simulink model "sysgenConcatenatedFEC"  (Simulink 7.4)
settings: Solver=ode45  SolverMode=SingleTasking  StartTime=0.0  StopTime=5000  RelTol=1e-3
undefined symbols (not defined in the file or in its folder): De, Interleaver, interleaver
libraries: xbsIndex_r4 x119, commchan3 x2, commdigbbndpm3 x2, xbsCopyrightNotice_r4 x1
(part 2 of 2)

== system sysgenConcatenatedFEC/Encoder1/rsenc ==
  note: The Outer Encoder is implemented by selecting  the RS Encoder block in the Xilinx Communication library. The
      | RS Encoder block has a pull down option to implement the DVB specifications specified in the standard. The
      | Reinterpret1 block at the input of the RS encoder converts the input FIX8_6 to UFIX8_0. The rfd output from the RS
      | Encoder block is used for handshaking to avoid any input data being dropped when the RS Encoder is generating
      | parity symbols.The RS Encoder block synchronizes its output to the first valid data received at the input.
  din : Inport  OutDataType=sfix(16)  OutScaling=2^0
  Constant : xbsIndex_r4/Constant  arith_type=Boolean  const=1  n_bits=1  bin_pt=0  explicit_period=on  period=1  equ=P=C  opselect=C  inp2=PCIN>>17  opr=+  inp1=P  carry=CIN  dbl_ovrd=off  block_type=constant
      settings: block_version=VER_STRING_GOES_HERE
  Delay : xbsIndex_r4/Delay  en=off  latency=2  dbl_ovrd=off  reg_retiming=off  block_type=delay
      settings: infoedit="Delay line having  configurable length.<P><P>Hardware notes: A delay line is a chain, each link of which is an SRL16 followed by a flip-flop. If register retiming is enabled, the delay line is a chain of flip-flops."  xl_area=[0, 0, 0, 0, 0, 0, 0]  block_version=VER_STRING_GOES_HERE
  RS Encoder : Subsystem
      settings: CopyFcn=set_param(gcb, 'LinkStatus', 'none');
  Reinterpret : xbsIndex_r4/Reinterpret  force_arith_type=on  arith_type=Unsigned  force_bin_pt=on  bin_pt=0  block_type=cast
      settings: infoedit="Changes type of samples without altering their binary representation.<P><P>Hardware notes: In hardware this block costs nothing.<P><P>Example:  Suppose the input is 6 bits wide, signed, with 2 fractional bits, and the output is forced to unsigned with 0 fractional bits.  Then an input of -2.0 (1110.00 in binary 2's complement) becomes an output of 56 (111000 in binary)."  block_version=VER_STRING_GOES_HERE
  tmt : Terminator
  dout : Outport  OutDataType=sfix(16)  OutScaling=2^0
  vout : Outport  Port=2  OutDataType=sfix(16)  OutScaling=2^0
  rfd : Outport  Port=3  OutDataType=sfix(16)  OutScaling=2^0
  wires:
  Constant/1 -> Delay/1
  Delay/1 -> RS Encoder/2(vin)
  RS Encoder/2(vout) -> vout/1
  RS Encoder/3(info) -> tmt/1
  RS Encoder/4(rfd) -> rfd/1
  Reinterpret/1 -> RS Encoder/1(din)
  din/1 -> Reinterpret/1
  RS Encoder/1(dout) -> dout/1

== system sysgenConcatenatedFEC/Decoder1/cvdeint/Rising Edge Detector1 ==
  Din : Inport  OutDataType=sfix(16)  OutScaling=2^0
  Delay : xbsIndex_r4/Delay  en=off  latency=1  dbl_ovrd=off  reg_retiming=off  block_type=delay
      settings: block_version=12.1
  Inverter2 : xbsIndex_r4/Inverter  en=off  latency=0  dbl_ovrd=off  block_type=inv
      settings: block_version=9.1
  Logical : xbsIndex_r4/Logical  logical_function=AND  inputs=2  en=off  latency=0  precision=Full  arith_type=Unsigned  n_bits=16  bin_pt=0  align_bp=on  dbl_ovrd=off  block_type=logical
      settings: block_version=9.1
  Register1 : xbsIndex_r4/Register  init=0  rst=off  en=off  dbl_ovrd=off  block_type=register
      settings: block_version=9.1
  Dout : Outport  OutDataType=sfix(16)  OutScaling=2^0
  wires:
  Delay/1 -> Dout/1
  Inverter2/1 -> Logical/2
  Register1/1 -> Inverter2/1
  Din/1 -> Logical/1, Register1/1
  Logical/1 -> Delay/1

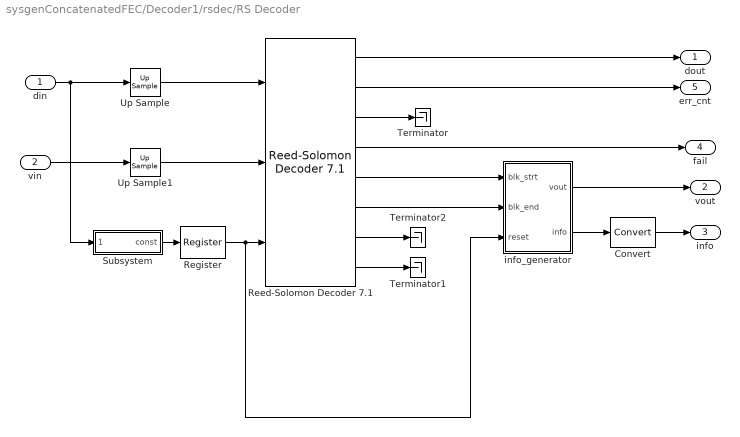
== system sysgenConcatenatedFEC/Decoder1/rsdec/RS Decoder ==
  din : Inport  OutDataType=sfix(16)  OutScaling=2^0
  vin : Inport  Port=2  OutDataType=sfix(16)  OutScaling=2^0
  Convert : xbsIndex_r4/Convert  arith_type=Boolean  n_bits=8  bin_pt=6  quantization=Truncate  overflow=Wrap  en=off  latency=0  dbl_ovrd=off  pipeline=off  block_type=convert
      settings: infoedit=The input is presented at the output after quantization and overflow effects.<P><P>Hardware notes: Additional hardware is used when rounding or saturation is selected and output width is less than the input width.  block_version=VER_STRING_GOES_HERE
  "Reed-Solomon Decoder 7.1 " : xbsIndex_r4/Reed-Solomon Decoder 7.1   code_specification=DVB  symbol_width=8  field_polynomial=285  scaling_factor=1  generator_start=0  variable_block_length=off  symbols_per_block=204  data_symbols=188  variable_number_of_check_symbols=off  define_supported_r_in_values=off  number_of_supported_r_in_values=2  supported_r_in_definition_file='no_coe_file_loaded'  optimization=Speed  self_recovering=off  memory_style=Automatic  clocks_per_symbol=8  number_of_channels=1  number_of_puncture_patterns=0  puncture_definition_file='no_coe_file_loaded'  clock_enable=off  info_end=off  synchronous_reset=on  original_delayed_data=off  erase=off  error_statistics=off  marker_bits=off  number_of_marker_bits=1  ip_name=Reed-Solomon Decoder  ip_version=7.1  dsptool_ready=false  ipcore_usecache=true  ipcore_useipmodelcache=true  wrapper_available=true  port_translation_map={ 'ce' => 'en', 'sr' => 'rst'}  structural_sim=true  ipcore_do_not_force_period=true  block_type=rs_decoder_v7_1
      settings: block_version=12.2
  Register : xbsIndex_r4/Register  init=0  rst=off  en=off  dbl_ovrd=off  block_type=register
      settings: block_version=12.1
  Subsystem : Subsystem
  Terminator : Terminator
  Terminator1 : Terminator
  Terminator2 : Terminator
  Up Sample : xbsIndex_r4/Up Sample  sample_ratio=8  copy_samples=on  en=off  latency=0  dbl_ovrd=off  block_type=usamp
      settings: block_version=12.1
  Up Sample1 : xbsIndex_r4/Up Sample  sample_ratio=8  copy_samples=on  en=off  latency=0  dbl_ovrd=off  block_type=usamp
      settings: block_version=12.1
  info_generator : Subsystem  mask{sym_width=8, kk=188}
      mask prompts: sym_width "Symbol Width"; kk "Number of information symbols per code block"
  dout : Outport  OutDataType=sfix(16)  OutScaling=2^0
  vout : Outport  Port=2  OutDataType=sfix(16)  OutScaling=2^0
  info : Outport  Port=3  OutDataType=sfix(16)  OutScaling=2^0
  fail : Outport  Port=4  OutDataType=sfix(16)  OutScaling=2^0
  err_cnt : Outport  Port=5  OutDataType=sfix(16)  OutScaling=2^0
  wires:
  "Reed-Solomon Decoder 7.1 "/7 -> Terminator2/1
  "Reed-Solomon Decoder 7.1 "/8 -> Terminator1/1
  "Reed-Solomon Decoder 7.1 "/3 -> Terminator/1
  "Reed-Solomon Decoder 7.1 "/4 -> fail/1
  "Reed-Solomon Decoder 7.1 "/2 -> err_cnt/1
  Convert/1 -> info/1
  Subsystem/1(const) -> Register/1
  din/1 -> Subsystem/1(sample), Up Sample/1
  vin/1 -> Up Sample1/1
  "Reed-Solomon Decoder 7.1 "/1 -> dout/1
  "Reed-Solomon Decoder 7.1 "/6 -> info_generator/2(blk_end)
  "Reed-Solomon Decoder 7.1 "/5 -> info_generator/1(blk_strt)
  info_generator/1(vout) -> vout/1
  info_generator/2(info) -> Convert/1
  Up Sample/1 -> "Reed-Solomon Decoder 7.1 "/1
  Up Sample1/1 -> "Reed-Solomon Decoder 7.1 "/2
  Register/1 -> info_generator/3(reset), "Reed-Solomon Decoder 7.1 "/3

== system sysgenConcatenatedFEC/Encoder1/int/Rising Edge Detector1 ==
  Din : Inport  OutDataType=sfix(16)  OutScaling=2^0
  Delay : xbsIndex_r4/Delay  en=off  latency=1  dbl_ovrd=off  reg_retiming=off  block_type=delay
      settings: block_version=12.1
  Inverter2 : xbsIndex_r4/Inverter  en=off  latency=0  dbl_ovrd=off  block_type=inv
      settings: block_version=9.1
  Logical : xbsIndex_r4/Logical  logical_function=AND  inputs=2  en=off  latency=0  precision=Full  arith_type=Unsigned  n_bits=16  bin_pt=0  align_bp=on  dbl_ovrd=off  block_type=logical
      settings: block_version=9.1
  Register1 : xbsIndex_r4/Register  init=0  rst=off  en=off  dbl_ovrd=off  block_type=register
      settings: block_version=9.1
  Dout : Outport  OutDataType=sfix(16)  OutScaling=2^0
  wires:
  Delay/1 -> Dout/1
  Inverter2/1 -> Logical/2
  Register1/1 -> Inverter2/1
  Din/1 -> Logical/1, Register1/1
  Logical/1 -> Delay/1

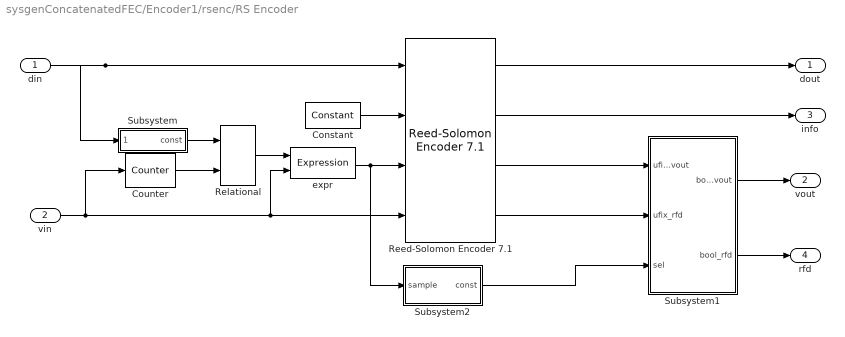
== system sysgenConcatenatedFEC/Encoder1/rsenc/RS Encoder ==
  din : Inport  OutDataType=sfix(16)  OutScaling=2^0
  vin : Inport  Port=2  OutDataType=sfix(16)  OutScaling=2^0
  Constant : xbsIndex_r4/Constant  arith_type=Boolean  const=0  n_bits=1  bin_pt=0  explicit_period=off  period=1  equ=P=C  opselect=C  inp2=PCIN>>17  opr=+  inp1=P  carry=CIN  dbl_ovrd=off  block_type=constant
      settings: block_version=VER_STRING_GOES_HERE
  Counter : xbsIndex_r4/Counter  cnt_type=Count Limited  cnt_to=204-1  operation=Up  start_count=0  cnt_by_val=1  arith_type=Unsigned  n_bits=8  bin_pt=0  load_pin=off  rst=off  en=on  explicit_period=off  period=1  dbl_ovrd=off  use_behavioral_HDL=off  implementation=Fabric  use_rpm=off  block_type=counter
      settings: infoedit="Configurable up, down and up/down counter.<P><P>Hardware notes: Free running counters are the least expensive in hardware.  A count limited counter is implemented by combining a counter with a comparator."  block_version=VER_STRING_GOES_HERE
  "Reed-Solomon Encoder 7.1 " : xbsIndex_r4/Reed-Solomon Encoder 7.1   code_specification=DVB  variable_number_of_check_symbols=off  variable_block_length=off  symbol_width=8  field_polynomial=285  scaling_factor=1  generator_start=0  symbol_per_block=204  data_symbols=188  check_symbol_generator=Fixed_Architecture  memory_style=Automatic  number_of_channels=1  ce=off  rdy=on  nd=on  rfd=on  sclr=off  rffd=off  ip_name=Reed-Solomon Encoder  ip_version=7.1  dsptool_ready=false  ipcore_usecache=true  ipcore_useipmodelcache=true  wrapper_available=true  port_translation_map={ 'ce' => 'en', 'sclr' => 'rst'}  structural_sim=false  ipcore_do_not_force_period=true  block_type=rs_encoder_v7_1
      settings: block_version=12.2
  Relational : xbsIndex_r4/Relational  mode=a=b  en=off  latency=0  dbl_ovrd=off  block_type=relational
      settings: block_version=VER_STRING_GOES_HERE
  Subsystem : Subsystem
  Subsystem1 : Subsystem
  Subsystem2 : Subsystem
  expr : xbsIndex_r4/Expression  expression=a & b  align_bp=on  en=off  latency=0  precision=Full  arith_type=Unsigned  n_bits=8  bin_pt=2  dbl_ovrd=off  block_type=expr
      settings: block_version=VER_STRING_GOES_HERE
  dout : Outport  OutDataType=sfix(16)  OutScaling=2^0
  vout : Outport  Port=2  OutDataType=sfix(16)  OutScaling=2^0
  info : Outport  Port=3  OutDataType=sfix(16)  OutScaling=2^0
  rfd : Outport  Port=4  OutDataType=sfix(16)  OutScaling=2^0
  wires:
  Subsystem2/1(const) -> Subsystem1/3(sel)
  din/1 -> Subsystem/1(sample), "Reed-Solomon Encoder 7.1 "/1
  "Reed-Solomon Encoder 7.1 "/1 -> dout/1
  "Reed-Solomon Encoder 7.1 "/2 -> info/1
  Constant/1 -> "Reed-Solomon Encoder 7.1 "/2
  vin/1 -> Counter/1, expr/2, "Reed-Solomon Encoder 7.1 "/4
  expr/1 -> Subsystem2/1(sample), "Reed-Solomon Encoder 7.1 "/3
  Relational/1 -> expr/1
  Counter/1 -> Relational/2
  "Reed-Solomon Encoder 7.1 "/3 -> Subsystem1/1(ufix_vout)
  "Reed-Solomon Encoder 7.1 "/4 -> Subsystem1/2(ufix_rfd)
  Subsystem1/2(bool_rfd) -> rfd/1
  Subsystem/1(const) -> Relational/1
  Subsystem1/1(bool_vout) -> vout/1

== system sysgenConcatenatedFEC/Decoder1/rsdec/RS Decoder/Subsystem ==
  sample : Inport  OutDataType=sfix(16)  OutScaling=2^0
  Constant4 : xbsIndex_r4/Constant  arith_type=Boolean  const=0  n_bits=1  bin_pt=0  explicit_period=off  period=1  equ=P=C  opselect=C  inp2=PCIN>>17  opr=+  inp1=P  carry=CIN  dbl_ovrd=off  block_type=constant
      settings: block_version=VER_STRING_GOES_HERE
  Slice : xbsIndex_r4/Slice  nbits=1  boolean_output=on  mode=Upper Bit Location + Width  bit1=0  base1=MSB of Input  bit0=0  base0=LSB of Input  dbl_ovrd=off  block_type=slice
      settings: infoedit="Extracts a given range of bits from each input sample and presents it at the output.  The output type is ordinarily unsigned with binary point at zero, but can be Boolean when the slice is one bit wide.<P><P>Hardware notes: In hardware this block costs nothing."  block_version=VER_STRING_GOES_HERE
  expr2 : xbsIndex_r4/Expression  expression=a & b  align_bp=on  en=off  latency=0  precision=Full  arith_type=Unsigned  n_bits=8  bin_pt=2  dbl_ovrd=off  block_type=expr
      settings: block_version=VER_STRING_GOES_HERE
  const : Outport  OutDataType=sfix(16)  OutScaling=2^0
  wires:
  expr2/1 -> const/1
  sample/1 -> Slice/1
  Slice/1 -> expr2/1
  Constant4/1 -> expr2/2

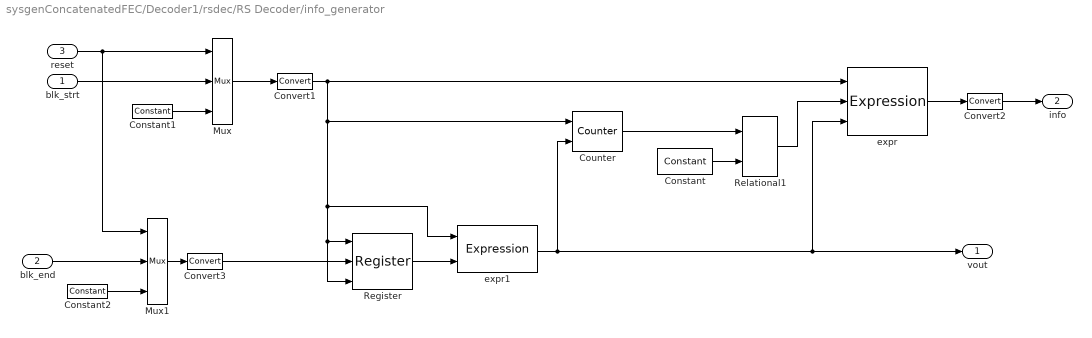
== system sysgenConcatenatedFEC/Decoder1/rsdec/RS Decoder/info_generator ==
  blk_strt : Inport  OutDataType=sfix(16)  OutScaling=2^0
  blk_end : Inport  Port=2  OutDataType=sfix(16)  OutScaling=2^0
  reset : Inport  Port=3  OutDataType=sfix(16)  OutScaling=2^0
  Constant : xbsIndex_r4/Constant  arith_type=Unsigned  const=kk-1  n_bits=8  bin_pt=0  explicit_period=off  period=1  equ=P=C  opselect=C  inp2=PCIN>>17  opr=+  inp1=P  carry=CIN  dbl_ovrd=off  block_type=constant
      settings: block_version=VER_STRING_GOES_HERE
  Constant1 : xbsIndex_r4/Constant  arith_type=Boolean  const=0  n_bits=1  bin_pt=0  explicit_period=off  period=1  equ=P=C  opselect=C  inp2=PCIN>>17  opr=+  inp1=P  carry=CIN  dbl_ovrd=off  block_type=constant
      settings: block_version=VER_STRING_GOES_HERE
  Constant2 : xbsIndex_r4/Constant  arith_type=Boolean  const=0  n_bits=1  bin_pt=0  explicit_period=off  period=1  equ=P=C  opselect=C  inp2=PCIN>>17  opr=+  inp1=P  carry=CIN  dbl_ovrd=off  block_type=constant
      settings: block_version=VER_STRING_GOES_HERE
  Convert1 : xbsIndex_r4/Convert  arith_type=Boolean  n_bits=1  bin_pt=0  quantization=Truncate  overflow=Wrap  en=off  latency=0  dbl_ovrd=off  pipeline=off  block_type=convert
      settings: infoedit=The input is presented at the output after quantization and overflow effects.<P><P>Hardware notes: Additional hardware is used when rounding or saturation is selected and output width is less than the input width.  block_version=VER_STRING_GOES_HERE
  Convert2 : xbsIndex_r4/Convert  arith_type=Unsigned  n_bits=1  bin_pt=0  quantization=Truncate  overflow=Wrap  en=off  latency=0  dbl_ovrd=off  pipeline=off  block_type=convert
      settings: infoedit=The input is presented at the output after quantization and overflow effects.<P><P>Hardware notes: Additional hardware is used when rounding or saturation is selected and output width is less than the input width.  block_version=VER_STRING_GOES_HERE
  Convert3 : xbsIndex_r4/Convert  arith_type=Boolean  n_bits=1  bin_pt=0  quantization=Truncate  overflow=Wrap  en=off  latency=0  dbl_ovrd=off  pipeline=off  block_type=convert
      settings: infoedit=The input is presented at the output after quantization and overflow effects.<P><P>Hardware notes: Additional hardware is used when rounding or saturation is selected and output width is less than the input width.  block_version=VER_STRING_GOES_HERE
  Counter : xbsIndex_r4/Counter  cnt_type=Free Running  cnt_to=inf  operation=Up  start_count=0  cnt_by_val=1  arith_type=Unsigned  n_bits=sym_width  bin_pt=0  load_pin=off  rst=on  en=on  explicit_period=off  period=1  dbl_ovrd=off  use_behavioral_HDL=off  implementation=Fabric  use_rpm=off  block_type=counter
      settings: infoedit="Configurable up, down and up/down counter.<P><P>Hardware notes: Free running counters are the least expensive in hardware.  A count limited counter is implemented by combining a counter with a comparator."  block_version=VER_STRING_GOES_HERE
  Mux : xbsIndex_r4/Mux  inputs=2  en=off  latency=0  precision=Full  arith_type=Unsigned  n_bits=8  bin_pt=2  quantization=Truncate  overflow=Wrap  dbl_ovrd=off  block_type=mux
      settings: block_version=VER_STRING_GOES_HERE
  Mux1 : xbsIndex_r4/Mux  inputs=2  en=off  latency=0  precision=Full  arith_type=Unsigned  n_bits=8  bin_pt=2  quantization=Truncate  overflow=Wrap  dbl_ovrd=off  block_type=mux
      settings: block_version=VER_STRING_GOES_HERE
  Register : xbsIndex_r4/Register  init=0  rst=on  en=on  dbl_ovrd=off  block_type=register
      settings: block_version=VER_STRING_GOES_HERE
  Relational1 : xbsIndex_r4/Relational  mode=a<b  en=off  latency=0  dbl_ovrd=off  block_type=relational
      settings: block_version=VER_STRING_GOES_HERE
  expr : xbsIndex_r4/Expression  expression=(a | b) & c  align_bp=on  en=off  latency=0  precision=Full  arith_type=Unsigned  n_bits=8  bin_pt=2  dbl_ovrd=off  block_type=expr
      settings: block_version=VER_STRING_GOES_HERE
  expr1 : xbsIndex_r4/Expression  expression=a | b  align_bp=on  en=off  latency=0  precision=Full  arith_type=Unsigned  n_bits=8  bin_pt=2  dbl_ovrd=off  block_type=expr
      settings: block_version=VER_STRING_GOES_HERE
  vout : Outport  OutDataType=sfix(16)  OutScaling=2^0
  info : Outport  Port=2  OutDataType=sfix(16)  OutScaling=2^0
  wires:
  Convert3/1 -> Register/2
  Constant/1 -> Relational1/2
  Relational1/1 -> expr/2
  Counter/1 -> Relational1/1
  Convert1/1 -> expr/1, Counter/1, Register/1, Register/3, expr1/1
  expr/1 -> Convert2/1
  Convert2/1 -> info/1
  Mux/1 -> Convert1/1
  Constant1/1 -> Mux/3
  blk_strt/1 -> Mux/2
  reset/1 -> Mux/1, Mux1/1
  Mux1/1 -> Convert3/1
  Constant2/1 -> Mux1/3
  blk_end/1 -> Mux1/2
  Register/1 -> expr1/2
  expr1/1 -> expr/3, vout/1, Counter/2

== system sysgenConcatenatedFEC/Encoder1/rsenc/RS Encoder/Subsystem ==
  sample : Inport  OutDataType=sfix(16)  OutScaling=2^0
  Constant4 : xbsIndex_r4/Constant  arith_type=Unsigned  const=0  n_bits=1  bin_pt=0  explicit_period=off  period=1  equ=P=C  opselect=C  inp2=PCIN>>17  opr=+  inp1=P  carry=CIN  dbl_ovrd=off  block_type=constant
      settings: block_version=VER_STRING_GOES_HERE
  Slice : xbsIndex_r4/Slice  nbits=1  boolean_output=off  mode=Upper Bit Location + Width  bit1=0  base1=MSB of Input  bit0=0  base0=LSB of Input  dbl_ovrd=off  block_type=slice
      settings: infoedit="Extracts a given range of bits from each input sample and presents it at the output.  The output type is ordinarily unsigned with binary point at zero, but can be Boolean when the slice is one bit wide.<P><P>Hardware notes: In hardware this block costs nothing."  block_version=VER_STRING_GOES_HERE
  expr2 : xbsIndex_r4/Expression  expression=a & b  align_bp=on  en=off  latency=0  precision=Full  arith_type=Unsigned  n_bits=8  bin_pt=2  dbl_ovrd=off  block_type=expr
      settings: block_version=VER_STRING_GOES_HERE
  const : Outport  OutDataType=sfix(16)  OutScaling=2^0
  wires:
  Constant4/1 -> expr2/2
  Slice/1 -> expr2/1
  sample/1 -> Slice/1
  expr2/1 -> const/1

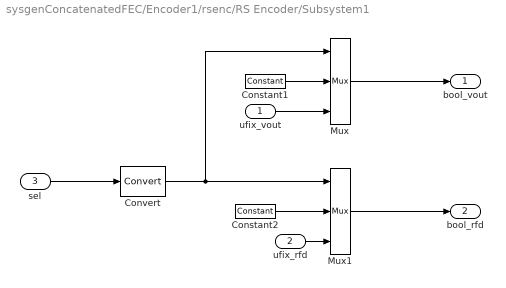
== system sysgenConcatenatedFEC/Encoder1/rsenc/RS Encoder/Subsystem1 ==
  ufix_vout : Inport  OutDataType=sfix(16)  OutScaling=2^0
  ufix_rfd : Inport  Port=2  OutDataType=sfix(16)  OutScaling=2^0
  sel : Inport  Port=3  OutDataType=sfix(16)  OutScaling=2^0
  Constant1 : xbsIndex_r4/Constant  arith_type=Boolean  const=0  n_bits=1  bin_pt=0  explicit_period=off  period=1  equ=P=C  opselect=C  inp2=PCIN>>17  opr=+  inp1=P  carry=CIN  dbl_ovrd=off  block_type=constant
      settings: block_version=VER_STRING_GOES_HERE
  Constant2 : xbsIndex_r4/Constant  arith_type=Boolean  const=1  n_bits=1  bin_pt=0  explicit_period=off  period=1  equ=P=C  opselect=C  inp2=PCIN>>17  opr=+  inp1=P  carry=CIN  dbl_ovrd=off  block_type=constant
      settings: block_version=VER_STRING_GOES_HERE
  Convert : xbsIndex_r4/Convert  arith_type=Boolean  n_bits=16  bin_pt=14  quantization=Truncate  overflow=Wrap  en=off  latency=0  dbl_ovrd=off  pipeline=off  block_type=convert
      settings: block_version=12.1
  Mux : xbsIndex_r4/Mux  inputs=2  en=off  latency=0  precision=Full  arith_type=Unsigned  n_bits=8  bin_pt=2  quantization=Truncate  overflow=Wrap  dbl_ovrd=off  block_type=mux
      settings: block_version=VER_STRING_GOES_HERE
  Mux1 : xbsIndex_r4/Mux  inputs=2  en=off  latency=0  precision=Full  arith_type=Unsigned  n_bits=8  bin_pt=2  quantization=Truncate  overflow=Wrap  dbl_ovrd=off  block_type=mux
      settings: block_version=VER_STRING_GOES_HERE
  bool_vout : Outport  OutDataType=sfix(16)  OutScaling=2^0
  bool_rfd : Outport  Port=2  OutDataType=sfix(16)  OutScaling=2^0
  wires:
  Mux/1 -> bool_vout/1
  Mux1/1 -> bool_rfd/1
  Constant1/1 -> Mux/2
  Constant2/1 -> Mux1/2
  sel/1 -> Convert/1
  ufix_vout/1 -> Mux/3
  ufix_rfd/1 -> Mux1/3
  Convert/1 -> Mux/1, Mux1/1

== system sysgenConcatenatedFEC/Encoder1/rsenc/RS Encoder/Subsystem2 ==
  sample : Inport  OutDataType=sfix(16)  OutScaling=2^0
  Constant3 : xbsIndex_r4/Constant  arith_type=Unsigned  const=1  n_bits=1  bin_pt=0  explicit_period=off  period=1  equ=P=C  opselect=C  inp2=PCIN>>17  opr=+  inp1=P  carry=CIN  dbl_ovrd=off  block_type=constant
      settings: block_version=VER_STRING_GOES_HERE
  Convert2 : xbsIndex_r4/Convert  arith_type=Unsigned  n_bits=1  bin_pt=0  quantization=Truncate  overflow=Wrap  en=off  latency=0  dbl_ovrd=off  pipeline=off  block_type=convert
      settings: infoedit=The input is presented at the output after quantization and overflow effects.<P><P>Hardware notes: Additional hardware is used when rounding or saturation is selected and output width is less than the input width.  block_version=VER_STRING_GOES_HERE
  expr1 : xbsIndex_r4/Expression  expression=a | b  align_bp=on  en=off  latency=0  precision=Full  arith_type=Unsigned  n_bits=8  bin_pt=2  dbl_ovrd=off  block_type=expr
      settings: block_version=VER_STRING_GOES_HERE
  const : Outport  OutDataType=sfix(16)  OutScaling=2^0
  wires:
  Constant3/1 -> expr1/2
  Convert2/1 -> expr1/1
  sample/1 -> Convert2/1
  expr1/1 -> const/1
